simulink model "santoso_part_A_section_c_R2025a"  (R2025a)
settings: Solver=VariableStepAuto  StartTime=0.0  StopTime=300  MaxStep=1  RelTol=1e-3  AbsTol=1e-3  EnableMultiTasking=on
libraries: fuzblock x1
settings Model: ExtModeTrigMode=oneshot  ExtModeArmWhenConnect=off  Creator=uos  LastModifiedBy=coa22ws
settings SolverCC: AutoScaleAbsTol=off  AlgebraicLoopSolver=TrustRegion
settings DataIOCC: SaveFormat=Array  SignalLoggingSaveFormat=ModelDataLogs  SaveOutput=off  SaveTime=off  ReturnWorkspaceOutputs=off  SignalLoggingName=sigsOut
settings OptimizationCC: BooleanDataType=off  ReuseModelBlockBuffer=off
settings DebuggingCC: SaveWithParameterizedLinksMsg=none  UnderspecifiedInitializationDetection=Classic  MergeDetectMultiDrivingBlocksExec=none  SignalResolutionControl=TryResolveAllWithWarning  MultiTaskDSMMsg=warning  MultiTaskCondExecSysMsg=none  UnconnectedInputMsg=warning  UnconnectedOutputMsg=warning  UnconnectedLineMsg=warning  ArithmeticOperatorsInVariantConditions=warning
settings HardwareCC: ProdBitPerPointer=32.0  ProdBitPerSizeT=32.0  ProdBitPerPtrDiffT=32.0  ProdLargestAtomicFloat=None  ProdIntDivRoundTo=Undefined  ProdEndianess=Unspecified  ProdWordSize=32.0  ProdHWDeviceType=32-bit Generic  TargetUnknown=on
settings ModelReferenceCC: EnableRefExpFcnMdlSchedulingChecks=on  PropagateSignalLabelsOutOfModel=off
settings SFSimCC: SimUseLocalCustomCode=off  CustomCodeUndefinedFunction=UseInterfaceOnly
settings RTWCC: RTWUseLocalCustomCode=off  GPUComputeCapability=3.5  DLArmComputeVersion=19.05
settings GRTTargetCC: TargetLangStandard=C89/C90 (ANSI)  CombineOutputUpdateFcns=off  GRTInterface=on
settings ConfigComp: CovMetricSettings=dw  CovSaveCumulativeToWorkspaceVar=on  CovSaveSingleToWorkspaceVar=on  CovExternalEMLEnable=off

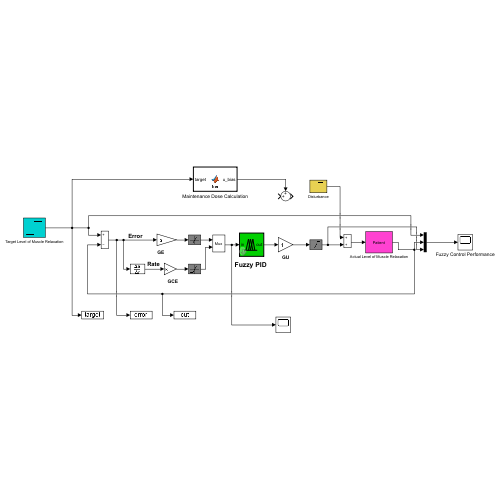
[thumbnail: Simulink's stored preview of the top-level diagram]
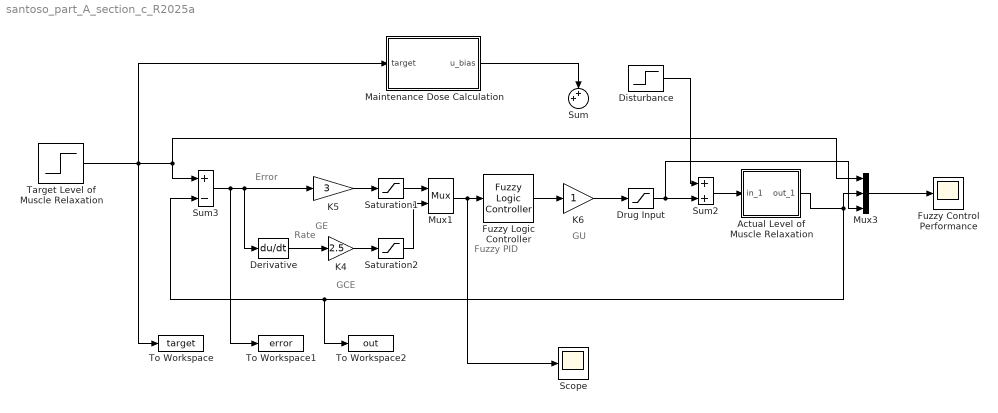
== system santoso_part_A_section_c_R2025a ==
  note: Fuzzy PID
  note: GE
  note: GCE
  note: GU
  note: Error
  note: Rate
  Actual Level of Muscle Relaxation : Subsystem
      mask Display: disp('Patient')
  Derivative : Derivative
  Disturbance : Step  Time=150  After=0.2  SampleTime=0
  Drug Input : Saturate  UpperLimit=1  LowerLimit=0
  Fuzzy Control Performance : Scope
      settings: ActiveDisplayYMinimum=-0.2318406887743647  ActiveDisplayYMaximum=1.9810963604437144
  Fuzzy Logic Controller : fuzblock/Fuzzy Logic  Controller  FIS="\"santoso_part_A_section_c.fis\""  OutputSampleNumber=101  DataType=double  UseLookupTable=off  NumBreakpoints=10  FuzzifiedInputs=off  RuleFiringStrengths=off  RuleOutputs=off  AggregatedOutputs=off  SimulateUsing=Interpreted execution  OutOfRangeInputValueMessage=warning  NoRuleFiredMessage=warning  EmptyOutputFuzzySetMessage=warning
  K4 : Gain  Gain=2.5  SaturateOnIntegerOverflow=on  OutDataTypeStr=Inherit: Same as input  ParamDataTypeStr=Inherit: Same as input
  K5 : Gain  Gain=3  SaturateOnIntegerOverflow=on  OutDataTypeStr=Inherit: Same as input  ParamDataTypeStr=Inherit: Same as input
  K6 : Gain  SaturateOnIntegerOverflow=on  OutDataTypeStr=Inherit: Same as input  ParamDataTypeStr=Inherit: Same as input
  Maintenance Dose Calculation : MATLAB Function  TreatAsAtomicUnit=on
  Mux1 : Mux  Inputs=2
  Mux3 : Mux  Inputs=3
  Saturation1 : Saturate  UpperLimit=1  LowerLimit=-1
  Saturation2 : Saturate  UpperLimit=1  LowerLimit=-1
  Scope : Scope
      settings: ActiveDisplayYMinimum=-0.54345492103180493  ActiveDisplayYMaximum=1.1714949912257562
  Sum : Sum  Inputs=++|
  Sum2 : Sum  InputSameDT=on  SaturateOnIntegerOverflow=on  OutDataTypeStr=Inherit: Same as first input
  Sum3 : Sum  Inputs=+-  InputSameDT=on  SaturateOnIntegerOverflow=on  OutDataTypeStr=Inherit: Same as first input
  Target Level of Muscle Relaxation : Step  Time=0  After=0.8  SampleTime=0
  To Workspace : ToWorkspace  VariableName=target  SaveFormat=Timeseries  SampleTime=-1
  To Workspace1 : ToWorkspace  VariableName=error  SaveFormat=Timeseries  SampleTime=-1
  To Workspace2 : ToWorkspace  VariableName=out  SaveFormat=Timeseries  SampleTime=-1
  wires:
  Saturation2/1 -> Mux1/2
  Saturation1/1 -> Mux1/1
  Mux1/1 -> Scope/1, Fuzzy Logic Controller/1
  Sum2/1 -> Actual Level of Muscle Relaxation/1(in_1)
  Drug Input/1 -> Mux3/3, Sum2/2
  Disturbance/1 -> Sum2/1
  Mux3/1 -> Fuzzy Control Performance/1
  K4/1 -> Saturation2/1
  Derivative/1 -> K4/1
  Sum3/1 -> K5/1, Derivative/1, To Workspace1/1
  K5/1 -> Saturation1/1
  Actual Level of Muscle Relaxation/1(out_1) -> Mux3/2, To Workspace2/1, Sum3/2
  Fuzzy Logic Controller/1 -> K6/1
  Target Level of Muscle Relaxation/1 -> To Workspace/1, Maintenance Dose Calculation/1(target), Mux3/1, Sum3/1
  Maintenance Dose Calculation/1(u_bias) -> Sum/1
  K6/1 -> Drug Input/1

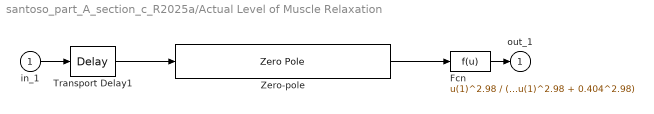
== system santoso_part_A_section_c_R2025a/Actual Level of Muscle Relaxation ==
  in_1 : Inport
  Fcn : Fcn  Expr=u(1)^2.98 / (u(1)^2.98 + 0.404^2.98)
  Transport Delay1 : TransportDelay
  Zero-pole : ZeroPole  Zeros=[-1/10.64]  Poles=[-1/20.0; -1/3.08; -1/4.81]  Gain=[10.64/(20.0*3.08*4.81)]
  out_1 : Outport  VectorParamsAs1DForOutWhenUnconnected=off
  wires:
  Fcn/1 -> out_1/1
  Zero-pole/1 -> Fcn/1
  in_1/1 -> Transport Delay1/1
  Transport Delay1/1 -> Zero-pole/1

== matlab function santoso_part_A_section_c_R2025a/Maintenance Dose Calculation ==
  data: target input; u_bias output
function u_bias = fcn(target)
    % Ensure target is within a safe range to avoid division by zero
    target = max(min(target, 0.99), 0.01); 
    u_bias = 0.404 * (target / (1 - target))^(1 / 2.98);
end
